simulink model "TwoBodySystem"  (R2022b)
settings: Solver=VariableStepAuto  StartTime=0.0  StopTime=10.0  RelTol=1e-3
values from neighbouring files (symbols this model uses):
  mu = 1.327e11    (= 132700000000)    [InitTwoBody.m]
  r0 = [2.029e8; -1.475e5; -1.1395e7]    [InitTwoBody.m]
  v0 = 0    [InitDamperMass.m]    (also in InitTwoBody.m = [3.021; 24.139; 10.964])
settings Model: Creator=filippocamaleonte  LastModifiedBy=filippocamaleonte

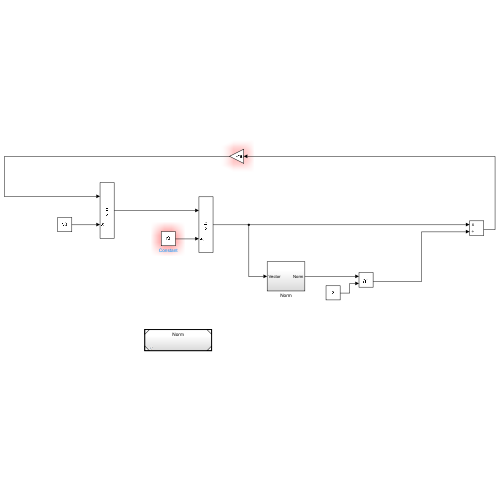
[thumbnail: Simulink's stored preview of the top-level diagram]
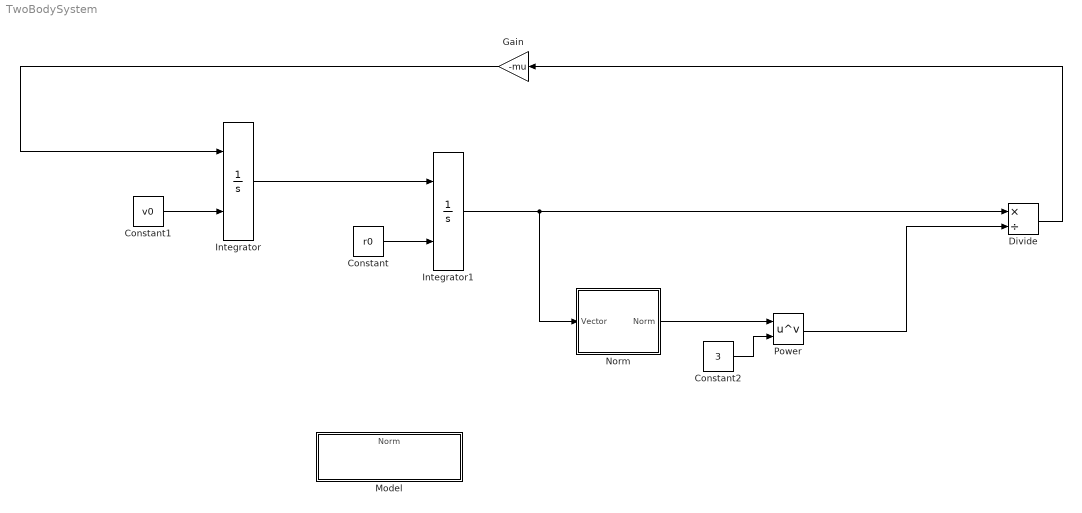
== system TwoBodySystem ==
  Constant : Constant  Value=r0
  Constant1 : Constant  Value=v0
  Constant2 : Constant  Value=3
  Divide : Product  Inputs=*/
  Gain : Gain  Gain=-mu
  Integrator : Integrator  InitialConditionSource=external
  Integrator1 : Integrator  InitialConditionSource=external
  Model : ModelReference  ModelNameDialog=Norm.slx  SimulationMode=Normal  ModelReferenceVersion=1.2
  Norm : Subsystem
  Power : Math  Operator=pow
  wires:
  Integrator/1 -> Integrator1/1
  Constant/1 -> Integrator1/2
  Constant1/1 -> Integrator/2
  Divide/1 -> Gain/1
  Integrator1/1 -> Divide/1, Norm/1(Vector)
  Norm/1(Norm) -> Power/1
  Constant2/1 -> Power/2
  Power/1 -> Divide/2
  Gain/1 -> Integrator/1

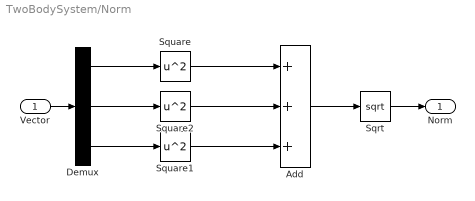
== system TwoBodySystem/Norm ==
  Vector : Inport
  Add : Sum  Inputs=+++
  Demux : Demux  Outputs=3
  Sqrt : Sqrt
  Square : Math  Operator=square
  Square1 : Math  Operator=square
  Square2 : Math  Operator=square
  Norm : Outport
  wires:
  Square/1 -> Add/1
  Add/1 -> Sqrt/1
  Demux/3 -> Square1/1
  Square2/1 -> Add/2
  Square1/1 -> Add/3
  Demux/1 -> Square/1
  Demux/2 -> Square2/1
  Vector/1 -> Demux/1
  Sqrt/1 -> Norm/1
